simulink model "modular_NL_Modell"  (R2016b)
settings: Solver=VariableStepAuto  StartTime=0.0  StopTime=15  RelTol=1e-3
values from neighbouring files (symbols this model uses):
  L_0 = 0.2    [StartSim.m]
  phi_0 = 0    [StartSim.m]
  r1 = 0.05    [StartSim.m]
  r2 = 0.05    [StartSim.m]
  T1 = 0.05    [StartSim.m]
  T2 = 0.05    [StartSim.m]
  ue1 = 6    [StartSim.m]
  ue2 = 3    [StartSim.m]
  x_0 = 0    [StartSim.m]
undefined symbols (not defined in the file or in its folder): K1, K2
libraries: simulink_extras x2
settings Model: Creator=Patrick  LastModifiedBy=Fritz

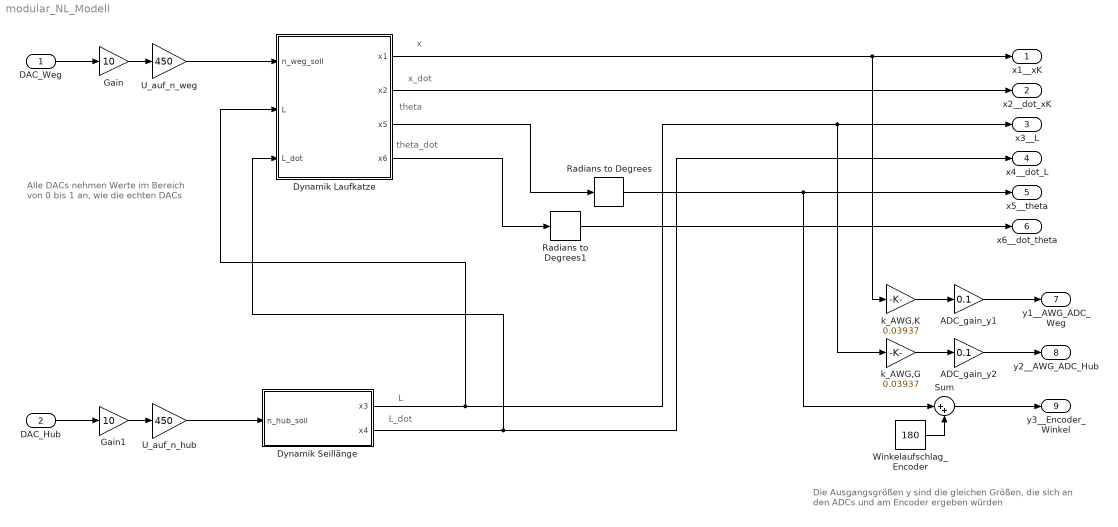
== system modular_NL_Modell ==
  note: Die Ausgangsgrößen y sind die gleichen Größen,
      | die sich an den ADCs und am Encoder ergeben würden
  note: Alle DACs nehmen Werte im Bereich
      | von 0 bis 1 an, wie die echten DACs
  note: L
  note: L_dot
  note: x
  note: x_dot
  note: theta
  note: theta_dot
  DAC_Weg : Inport
  DAC_Hub : Inport  Port=2
  ADC_gain_y1 : Gain  Gain=0.1
  ADC_gain_y2 : Gain  Gain=0.1
  Dynamik Laufkatze : Subsystem
  Dynamik Seillänge : Subsystem
  Gain : Gain  Gain=10
  Gain1 : Gain  Gain=10
  Radians to Degrees : simulink_extras/Transformations/Radians to Degrees
  Radians to Degrees1 : simulink_extras/Transformations/Radians to Degrees
  Sum : Sum  Inputs=|++
  U_auf_n_hub : Gain  Gain=450
  U_auf_n_weg : Gain  Gain=450
  Winkelaufschlag_Encoder : Constant  Value=180
  k_AWG,G : Gain  Gain=0.03937
  k_AWG,K : Gain  Gain=0.03937
  x1__xK : Outport  SignalName=x1__xK
  x2__dot_xK : Outport  Port=2  SignalName=x2__dot_xK
  x3__L : Outport  Port=3  SignalName=x3__L
  x4__dot_L : Outport  Port=4  SignalName=x4__dot_L
  x5__theta : Outport  Port=5  SignalName=x5__theta
  x6__dot_theta : Outport  Port=6  SignalName=x6__dot_theta
  y1__AWG_ADC_Weg : Outport  Port=7  SignalName=y1__AWG_ADC_Weg
  y2__AWG_ADC_Hub : Outport  Port=8  SignalName=y2__AWG_ADC_Hub
  y3__Encoder_Winkel : Outport  Port=9  SignalName=y3__Encoder_Winkel
  wires:
  Dynamik Laufkatze/1(x1) -> k_AWG,K/1, x1__xK/1
  Dynamik Laufkatze/2(x2) -> x2__dot_xK/1
  Dynamik Laufkatze/3(x5) -> Radians to Degrees/1
  Dynamik Laufkatze/4(x6) -> Radians to Degrees1/1
  Dynamik Seillänge/2(x4) -> x4__dot_L/1, Dynamik Laufkatze/3(L_dot)
  Radians to Degrees1/1 -> x6__dot_theta/1
  Radians to Degrees/1 -> Sum/1, x5__theta/1
  DAC_Weg/1 -> Gain/1
  Gain/1 -> U_auf_n_weg/1
  U_auf_n_weg/1 -> Dynamik Laufkatze/1(n_weg_soll)
  DAC_Hub/1 -> Gain1/1
  Gain1/1 -> U_auf_n_hub/1
  U_auf_n_hub/1 -> Dynamik Seillänge/1(n_hub_soll)
  k_AWG,K/1 -> ADC_gain_y1/1
  Dynamik Seillänge/1(x3) -> k_AWG,G/1, x3__L/1, Dynamik Laufkatze/2(L)
  k_AWG,G/1 -> ADC_gain_y2/1
  Winkelaufschlag_Encoder/1 -> Sum/2
  Sum/1 -> y3__Encoder_Winkel/1
  ADC_gain_y2/1 -> y2__AWG_ADC_Hub/1
  ADC_gain_y1/1 -> y1__AWG_ADC_Weg/1

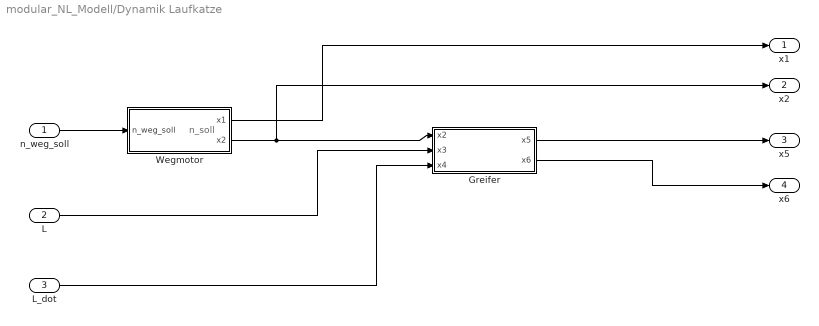
== system modular_NL_Modell/Dynamik Laufkatze ==
  note: n_soll
  n_weg_soll : Inport
  L : Inport  Port=2
  L_dot : Inport  Port=3
  Greifer : Subsystem
  Wegmotor : Subsystem
  x1 : Outport
  x2 : Outport  Port=2
  x5 : Outport  Port=3
  x6 : Outport  Port=4
  wires:
  n_weg_soll/1 -> Wegmotor/1(n_weg_soll)
  Wegmotor/1(x1) -> x1/1
  Wegmotor/2(x2) -> x2/1, Greifer/1(x2)
  Greifer/1(x5) -> x5/1
  Greifer/2(x6) -> x6/1
  L/1 -> Greifer/2(x3)
  L_dot/1 -> Greifer/3(x4)

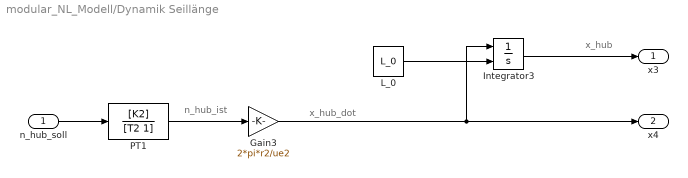
== system modular_NL_Modell/Dynamik Seillänge ==
  note: n_hub_ist
  note: x_hub_dot
  note: x_hub
  n_hub_soll : Inport
  Gain3 : Gain  Gain=2*pi*r2/ue2
  Integrator3 : Integrator  InitialConditionSource=external
  L_0 : Constant  Value=L_0
  PT1 : TransferFcn  Numerator=[K2]  Denominator=[T2 1]
  x3 : Outport
  x4 : Outport  Port=2
  wires:
  n_hub_soll/1 -> PT1/1
  PT1/1 -> Gain3/1
  Integrator3/1 -> x3/1
  L_0/1 -> Integrator3/2
  Gain3/1 -> Integrator3/1, x4/1

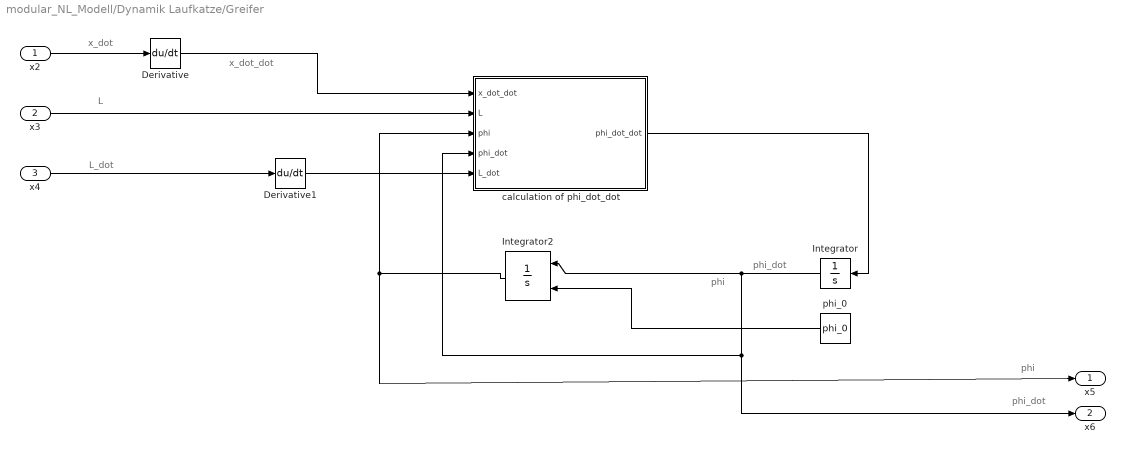
== system modular_NL_Modell/Dynamik Laufkatze/Greifer ==
  note: phi
  note: phi
  note: x_dot
  note: L
  note: phi_dot
  note: phi_dot
  note: x_dot_dot
  note: L_dot
  x2 : Inport
  x3 : Inport  Port=2
  x4 : Inport  Port=3
  Derivative : Derivative
  Derivative1 : Derivative
  Integrator : Integrator
  Integrator2 : Integrator  InitialConditionSource=external
  calculation of phi_dot_dot : MATLAB Function  TreatAsAtomicUnit=on
  phi_0 : Constant  Value=phi_0
  x5 : Outport
  x6 : Outport  Port=2
  wires:
  Derivative/1 -> calculation of phi_dot_dot/1(x_dot_dot)
  x2/1 -> Derivative/1
  Integrator/1 -> x6/1, calculation of phi_dot_dot/4(phi_dot), Integrator2/1
  x3/1 -> calculation of phi_dot_dot/2(L)
  calculation of phi_dot_dot/1(phi_dot_dot) -> Integrator/1
  Integrator2/1 -> x5/1, calculation of phi_dot_dot/3(phi)
  Derivative1/1 -> calculation of phi_dot_dot/5(L_dot)
  phi_0/1 -> Integrator2/2
  x4/1 -> Derivative1/1

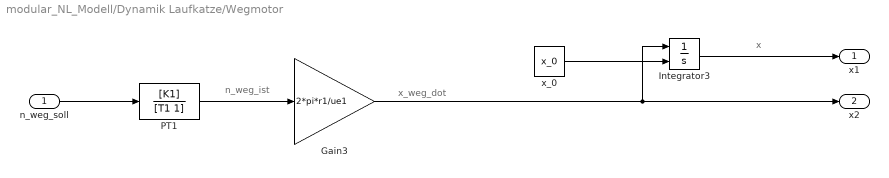
== system modular_NL_Modell/Dynamik Laufkatze/Wegmotor ==
  note: n_weg_ist
  note: x
  note: x_weg_dot
  n_weg_soll : Inport
  Gain3 : Gain  Gain=2*pi*r1/ue1
  Integrator3 : Integrator  InitialConditionSource=external
  PT1 : TransferFcn  Numerator=[K1]  Denominator=[T1 1]
  x_0 : Constant  Value=x_0
  x1 : Outport
  x2 : Outport  Port=2
  wires:
  x_0/1 -> Integrator3/2
  n_weg_soll/1 -> PT1/1
  PT1/1 -> Gain3/1
  Integrator3/1 -> x1/1
  Gain3/1 -> Integrator3/1, x2/1

== matlab function modular_NL_Modell/Dynamik Laufkatze/Greifer/calculation of phi_dot_dot ==
  data: x_dot_dot input; phi_dot_dot output; L input; phi input; phi_dot input; L_dot input
function phi_dot_dot = fcn(x_dot_dot,L,phi,phi_dot,L_dot)

phi_dot_dot = -(cos(phi)/L)*x_dot_dot-9.81/L*sin(phi)-2*L_dot*phi_dot;
